simulink model "zoomLensSim"  (Simulink 6.1)
settings: Solver=ode45  StartTime=0.0  StopTime=1/testFreq*5  RelTol=1e-3
undefined symbols (not defined in the file or in its folder): C1, testFreq, Tzoom, zoomRateLimit
settings Model: LastModifiedBy=Big E
settings DebuggingCC: SolverPrmCheckMsg=warning

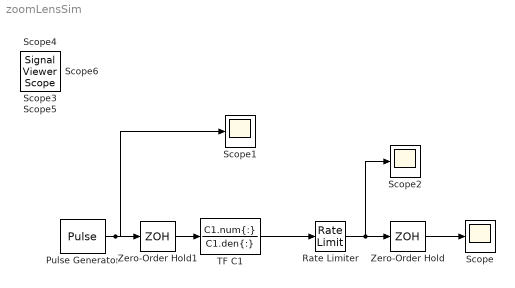
== system zoomLensSim ==
  Pulse Generator : DiscretePulseGenerator  PulseType=Time based  Amplitude=5000  Period=1/testFreq*2  PulseWidth=50
  Rate Limiter : RateLimiter  RisingSlewLimit=zoomRateLimit  FallingSlewLimit=-zoomRateLimit  SampleTimeMode=inherited
  Scope : Scope
  Scope1 : Scope
  Scope2 : Scope
      settings: SaveName=ScopeData2
  TF C1 : TransferFcn  Numerator=C1.num{:}  Denominator=C1.den{:}
  Zero-Order Hold : ZeroOrderHold  SampleTime=.033
  Zero-Order Hold1 : ZeroOrderHold  SampleTime=Tzoom
  Scope{3..6} (4 alike) : SignalViewerScope  IOType=viewer  RefreshTime=0.035000
  wires:
  TF C1/1 -> Rate Limiter/1
  Pulse Generator/1 -> Scope1/1, Zero-Order Hold1/1
  Rate Limiter/1 -> Zero-Order Hold/1, Scope2/1
  Zero-Order Hold/1 -> Scope/1
  Zero-Order Hold1/1 -> TF C1/1
